simulink model "oven_model_V3"  (R2026a)
settings: Solver=ode15s  StopTime=ovenV3_p.sim.warmupSeconds+ovenV3_p.sim.bakeSeconds+ovenV3_p.sim.recoverySeconds  MaxStep=2  RelTol=1e-05  AbsTol=1e-07
PreLoadFcn:
  | addpath(fileparts(get_param(bdroot,'FileName')));
InitFcn:
  | oven_refresh_model(bdroot);
model workspace (MAT data in the model file):
  ovenV3_g.eaveHeight = 0.15
  ovenV3_g.frontArea = 0.3239
  ovenV3_g.rearArea = 0.091
  ovenV3_g.plateArea = 0.0804247719319
  ovenV3_g.gapArea = 0.0020169024836
  ovenV3_g.fixedArea = 0.161033553653
  ovenV3_g.pizzaArea = 0.0706858347058
  ovenV3_g.totalArea = 0.4149
  ovenV3_g.frontRoofArea = 0.337253346962
  ovenV3_g.rearRoofArea = 0.0994971291643
  ovenV3_g.mouthArea = 0.078
  ovenV3_g.hatchArea = 0.02
  ovenV3_g.frontShellArea = 0.553420013629
  ovenV3_g.rearShellArea = 0.269394098784
  ovenV3_g.volume = [0.0701783333333 0.0197166666667]
  ovenV3_g.chimneyArea = 0.00785398163397
  ovenV3_g.inletArea = 0.0234
  ovenV3_g.roofMaterial.thickness = 0.002
  ovenV3_g.roofMaterial.rho = 7800
  ovenV3_g.roofMaterial.cp = 500
  ovenV3_g.roofMaterial.k = 45
  ovenV3_g.shellMass = [8.63335221261 4.20254794103]
  ovenV3_g.cordieriteMass = [4.18687239497 2.366 2.09104407023 2.09104407023]
  ovenV3_g.idx.gas = [1 2]
  ovenV3_g.idx.shell = [3 4]
  ovenV3_g.idx.fixed = 5
  ovenV3_g.idx.hearth = 6
  ovenV3_g.idx.plate = [7  15; 8  16; 9  17; 10  18; 11  19; 12  20; 13  21; 14  22]
  ovenV3_g.idx.base = [23  31; 24  32; 25  33; 26  34; 27  35; 28  36; 29  37; 30  38]
  ovenV3_g.idx.top = [39  47; 40  48; 41  49; 42  50; 43  51; 44  52; 45  53; 46  54]
  ovenV3_g.idx.water = [55  63; 56  64; 57  65; 58  66; 59  67; 60  68; 61  69; 62  70]
  ovenV3_g.idx.plateBottom = [71  79; 72  80; 73  81; 74  82; 75  83; 76  84; 77  85; 78  86]
  ovenV3_g.idx.shellOuter = [87 88]
  ovenV3_g.idx.fixedBottom = 89
  ovenV3_g.idx.hearthBottom = 90
  ovenV3_g.nStates = 90
  ovenV3_g.C = [91.410405836; 25.6818367739; 2158.33805315; 1050.63698526; 1884.09257774; 1064.7; 117.62122895; 117.62122895; 117.62122895; 117.62122895; 117.62122895; 117.62122895; 117.62122895; 117.62122895; 117.62122895; 117.62122895; 117.62122895; 117.62122895; 117.62122895; 117.62122895; 117.62122895; 117.62122895; 31.25; 31.25; 31.25; 31.25; 31.25; 31.25; 31.25; 31.25; 31.25; 31.25; 31.25; 31.25; 31.25; 31.25; 31.25; 31.25; 46.875; 46.875; 46.875; 46.875; 46.875; 46.875; 46.875; 46.875; 46.875; 46.875; 46.875; 46.875; 46.875; 46.875; 46.875; 46.875; 0; 0; 0; 0; 0; 0; 0; 0; 0; 0; 0; 0; 0; 0; 0; 0; 117.62122895; 117.62122895; 117.62122895; 117.62122895; 117.62122895; 117.62122895; 117.62122895; 117.62122895; 117.62122895; 117.62122895; 117.62122895; 117.62122895; 117.62122895; 117.62122895; 117.62122895; 117.62122895; 2158.33805315; 1050.63698526; 1884.09257774; 1064.7]
  ovenV3_g.shellU = 0.990980079298
  ovenV3_g.floorU = 0.990009900099
  ovenV3_g.shellThroughG = [24903.9006133; 12122.7344453]
  ovenV3_g.floorThroughG = [80.5167768263; 45.5; 5.02654824574; 5.02654824574; 5.02654824574; 5.02654824574; 5.02654824574; 5.02654824574; 5.02654824574; 5.02654824574; 5.02654824574; 5.02654824574; 5.02654824574; 5.02654824574; 5.02654824574; 5.02654824574; 5.02654824574; 5.02654824574]
  ovenV3_g.sectorConductance = 0.0318309886184
  ovenV3_g.labels = {'gas_front', 'gas_rear', 'shell_front', 'shell_rear', 'floor_fixed', 'hearth', 'plate_1_sector_1', 'plate_1_sector_2', 'plate_1_sector_3', 'plate_1_sector_4', 'plate_1_sector_5', 'plate_1_sector_6', 'plate_1_sector_7', 'plate_1_sector_8', 'plate_2_sector_1', 'plate_2_sector_2', 'plate_2_sector_3', 'plate_2_sector_4', 'plate_2_sector_5', 'plate_2_sector_6', 'plate_2_sector_7', 'plate_2_sector_8', 'base_1_sector_1', 'base_1_sector_2', 'base_1_sector_3', 'base_1_sector_4', 'base_1_sector_5', 'base_1_sector_6', 'base_1_sector_7', 'base_1_sector_8', 'base_2_sector_1', 'base_2_sector_2', 'base_2_sector_3', 'base_2_sector_4', 'base_2_sector_5', 'base_2_sector_6', 'base_2_sector_7', 'base_2_sector_8', 'top_1_sector_1', 'top_1_sector_2', 'top_1_sector_3', 'top_1_sector_4', 'top_1_sector_5', 'top_1_sector_6', 'top_1_sector_7', 'top_1_sector_8', 'top_2_sector_1', 'top_2_sector_2', 'top_2_sector_3', 'top_2_sector_4', 'top_2_sector_5', 'top_2_sector_6', 'top_2_sector_7', 'top_2_sector_8', 'water_1_sector_1', 'water_1_sector_2', 'water_1_sector_3', 'water_1_sector_4', 'water_1_sector_5', 'water_1_sector_6', 'water_1_sector_7', 'water_1_sector_8', 'water_2_sector_1', 'water_2_sector_2', 'water_2_sector_3', 'water_2_sector_4', 'water_2_sector_5', 'water_2_sector_6', 'water_2_sector_7', 'water_2_sector_8', 'plate_bottom_1_sector_1', 'plate_bottom_1_sector_2', 'plate_bottom_1_sector_3', 'plate_bottom_1_sector_4', 'plate_bottom_1_sector_5', 'plate_bottom_1_sector_6', 'plate_bottom_1_sector_7', 'plate_bottom_1_sector_8', 'plate_bottom_2_sector_1', 'plate_bottom_2_sector_2', 'plate_bottom_2_sector_3', 'plate_bottom_2_sector_4', 'plate_bottom_2_sector_5', 'plate_bottom_2_sector_6', 'plate_bottom_2_sector_7', 'plate_bottom_2_sector_8', 'shell_outer_front', 'shell_outer_rear', 'floor_fixed_bottom', 'hearth_bottom'}
  ovenV3_g.y0 = [298.15; 298.15; 298.15; 298.15; 298.15; 298.15; 298.15; 298.15; 298.15; 298.15; 298.15; 298.15; 298.15; 298.15; 298.15; 298.15; 298.15; 298.15; 298.15; 298.15; 298.15; 298.15; 298.15; 298.15; 298.15; 298.15; 298.15; 298.15; 298.15; 298.15; 298.15; 298.15; 298.15; 298.15; 298.15; 298.15; 298.15; 298.15; 298.15; 298.15; 298.15; 298.15; 298.15; 298.15; 298.15; 298.15; 298.15; 298.15; 298.15; 298.15; 298.15; 298.15; 298.15; 298.15; 0.015625; 0.015625; 0.015625; 0.015625; 0.015625; 0.015625; 0.015625; 0.015625; 0.015625; 0.015625; 0.015625; 0.015625; 0.015625; 0.015625; 0.015625; 0.015625; 298.15; 298.15; 298.15; 298.15; 298.15; 298.15; 298.15; 298.15; 298.15; 298.15; 298.15; 298.15; 298.15; 298.15; 298.15; 298.15; 298.15; 298.15; 298.15; 298.15]
  ovenV3_p.version = '3.0'
  ovenV3_p.ambient = 298.15
  ovenV3_p.sigma = 5.670374419e-08
  ovenV3_p.geom.width = 0.79
  ovenV3_p.geom.frontDepth = 0.41
  ovenV3_p.geom.rearWidth = 0.51
  ovenV3_p.geom.rearDepth = 0.14
  ovenV3_p.geom.plateDiameter = 0.32
  ovenV3_p.geom.plateCenters = [0.21  0.205; 0.58  0.205]
  ovenV3_p.geom.plateClearance = 0.001
  ovenV3_p.geom.roofShape = 'barrel'
  ovenV3_p.geom.height = 0.25
  ovenV3_p.geom.rise = 0.1
  ovenV3_p.geom.mouthWidth = 0.6
  ovenV3_p.geom.mouthHeight = 0.13
  ovenV3_p.geom.hatchWidth = 0.2
  ovenV3_p.geom.hatchHeight = 0.1
  ovenV3_p.geom.hatchOpenFraction = 0
  ovenV3_p.geom.sectors = 8
  ovenV3_p.floor.thickness = 0.01
  ovenV3_p.floor.rho = 2600
  ovenV3_p.floor.cp = 900
  ovenV3_p.floor.k = 2.5
  ovenV3_p.floor.emissivity = 0.85
  ovenV3_p.roof.material = 'steel'
  ovenV3_p.roof.steel.thickness = 0.002
  ovenV3_p.roof.steel.rho = 7800
  ovenV3_p.roof.steel.cp = 500
  ovenV3_p.roof.steel.k = 45
  ovenV3_p.roof.refractory.thickness = 0.03
  ovenV3_p.roof.refractory.rho = 2100
  ovenV3_p.roof.refractory.cp = 900
  ovenV3_p.roof.refractory.k = 1.3
  ovenV3_p.roof.emissivity = 0.8
  ovenV3_p.insulation.thickness = 0.05
  ovenV3_p.insulation.k = 0.055
  ovenV3_p.insulation.outsideH = 10
  ovenV3_p.flow.chimneyDiameter = 0.1
  ovenV3_p.flow.chimneyHeight = 0.5
  ovenV3_p.flow.chimneyPosition = 'front'
  ovenV3_p.flow.chimneyLoss = 3
  ovenV3_p.flow.inletLoss = 2
  ovenV3_p.flow.inletFraction = 0.3
  ovenV3_p.flow.mixingKgS = 0.012
  ovenV3_p.flow.cp = 1100
  ovenV3_p.flow.pressure = 101325
  ovenV3_p.flow.gasConstant = 287
  ovenV3_p.flow.gravity = 9.81
  ovenV3_p.fuel.kgH = 3.5
  ovenV3_p.fuel.lhv = 15000000
  ovenV3_p.fuel.efficiency = 0.7
  ovenV3_p.fuel.radiantFraction = 0.35
  ovenV3_p.fuel.radiantWeights = [0.15 0.6 0.25]
  ovenV3_p.heat.gasH = 18
  ovenV3_p.heat.pizzaH = 12
  ovenV3_p.heat.contactH = 150
  ovenV3_p.heat.pizzaInternalH = 90
  ovenV3_p.heat.shellLink = 1.5
  ovenV3_p.heat.rearExposureMean = 0.18
  ovenV3_p.heat.rearExposureAmplitude = 0.12
  ovenV3_p.heat.openingEmissivity = 0.8
  ovenV3_p.rotation.rpm = [2 2]
  ovenV3_p.rotation.initialPhase = [0 0]
  ovenV3_p.pizza.diameter = 0.3
  ovenV3_p.pizza.mass = 0.25
  ovenV3_p.pizza.cp = 2500
  ovenV3_p.pizza.baseMassFraction = 0.4
  ovenV3_p.pizza.waterFraction = 0.5
  ovenV3_p.pizza.initialTemperature = 298.15
  ovenV3_p.pizza.emissivity = 0.9
  ovenV3_p.pizza.latentHeat = 2260000
  ovenV3_p.pizza.evaporationTemperature = 373.15
  ovenV3_p.pizza.evaporationTransitionK = 2
  ovenV3_p.pizza.waterTransitionKg = 1e-05
  ovenV3_p.sim.warmupSeconds = 1800
  ovenV3_p.sim.bakeSeconds = 90
  ovenV3_p.sim.recoverySeconds = 90
  ovenV3_p.sim.outputStep = 5
  ovenV3_p.sim.maxStep = 2
  ovenV3_p.sim.relTol = 1e-05
  ovenV3_p.sim.absTol = 1e-07
settings Model: Creator=samue  LastModifiedBy=samue

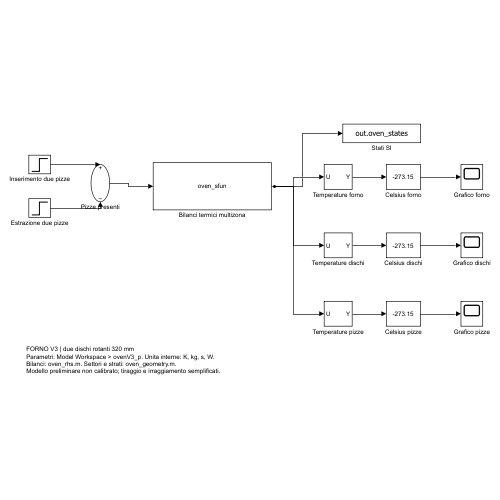
[thumbnail: Simulink's stored preview of the top-level diagram]
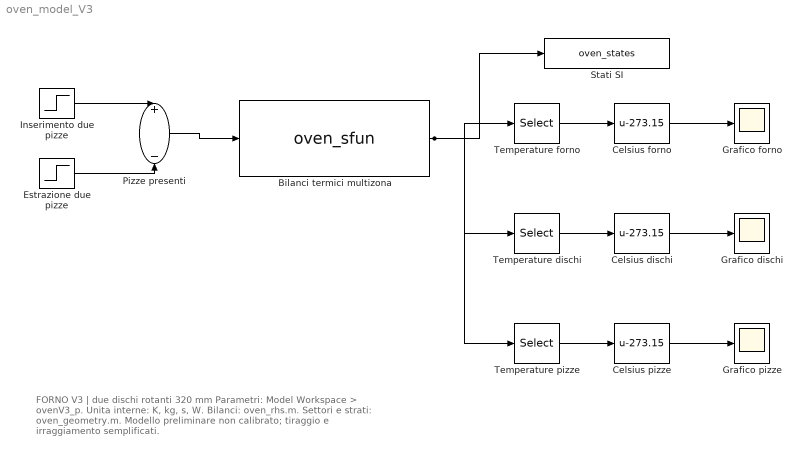
== system oven_model_V3 ==
  note: FORNO V3 | due dischi rotanti 320 mm
      | Parametri: Model Workspace > ovenV3_p. Unita interne: K, kg, s, W.
      | Bilanci: oven_rhs.m. Settori e strati: oven_geometry.m.
      | Modello preliminare non calibrato; tiraggio e irraggiamento semplificati.
  Bilanci termici multizona : M-S-Function  FunctionName=oven_sfun  Parameters=ovenV3_p,ovenV3_g
  Celsius dischi : Bias  Bias=-273.15  SaturateOnIntegerOverflow=off
  Celsius forno : Bias  Bias=-273.15  SaturateOnIntegerOverflow=off
  Celsius pizze : Bias  Bias=-273.15  SaturateOnIntegerOverflow=off
  Estrazione due pizze : Step  Time=ovenV3_p.sim.warmupSeconds+ovenV3_p.sim.bakeSeconds  SampleTime=0
  Grafico dischi : Scope
  Grafico forno : Scope
  Grafico pizze : Scope
  Inserimento due pizze : Step  Time=ovenV3_p.sim.warmupSeconds  SampleTime=0
  Pizze presenti : Sum  Inputs=+-
  Stati SI : ToWorkspace  VariableName=oven_states  SaveFormat=Structure With Time  SampleTime=-1
  Temperature dischi : Selector  IndexOptions=Index vector (dialog)  Indices=[7 8 9 10 11 12 13 14 15 16 17 18 19 20 21 22]  OutputSizes=1
  Temperature forno : Selector  IndexOptions=Index vector (dialog)  Indices=[1 2 3 4 5 6]  OutputSizes=1
  Temperature pizze : Selector  IndexOptions=Index vector (dialog)  Indices=[23 24 25 26 27 28 29 30 31 32 33 34 35 36 37 38 39 40 41 42 43 44 45 46 47 48 49 50 51 52 53 54]  OutputSizes=1
  wires:
  Inserimento due pizze/1 -> Pizze presenti/1
  Estrazione due pizze/1 -> Pizze presenti/2
  Pizze presenti/1 -> Bilanci termici multizona/1
  Bilanci termici multizona/1 -> Stati SI/1, Temperature forno/1, Temperature dischi/1, Temperature pizze/1
  Temperature forno/1 -> Celsius forno/1
  Celsius forno/1 -> Grafico forno/1
  Temperature dischi/1 -> Celsius dischi/1
  Celsius dischi/1 -> Grafico dischi/1
  Temperature pizze/1 -> Celsius pizze/1
  Celsius pizze/1 -> Grafico pizze/1
